simulink model "SecondaryPath_ANC"  (R2020a)
settings: Solver=FixedStepDiscrete  StartTime=0.0  StopTime=3  FixedStep=0.00025  RelTol=1e-3
libraries: dspsrcs4 x1, dspadpt3 x1
settings Model: Creator=The MathWorks, Inc.  LastModifiedBy=bruno
settings DataIOCC: ReturnWorkspaceOutputs=off
settings DebuggingCC: ArithmeticOperatorsInVariantConditions=warning
settings SFSimCC: CustomCodeUndefinedFunction=UseInterfaceOnly

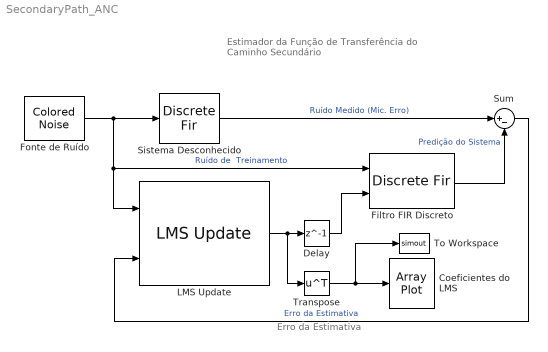
== system SecondaryPath_ANC ==
  note: Erro da Estimativa
  note: Estimador da Função de Transferência do
      | Caminho Secundário
  Coeficientes do LMS : ArrayPlot
  Delay : Delay  DelayLength=1
  Filtro FIR Discreto : DiscreteFir  CoefSource=Input port
      settings: InputPortMap=u0,u1
  Fonte de Ruído : dspsrcs4/Colored Noise  Color=white  InverseFrequencyPower=1  BoundedOutput=off  NumChannels=1  OutputDataType=double  SamplesPerFrame=1  SampleTime=1/4000  RandomStream=mt19937ar with seed  Seed=67  SimulateUsing=Interpreted execution
      settings: SourceProductBaseCode=DS
  LMS Update : dspadpt3/LMS Update  Method=Normalized LMS  Length=30  StepSizeSource=Property  StepSize=0.2  LeakageFactor=1.0  InitialConditions=0  EnableAdaptInput=off  EnableResetInput=off  SimulateUsing=Interpreted execution
      settings: SourceProductBaseCode=DS
  Sistema Desconhecido : DiscreteFir  Coefficients=[0.5 0.5 -.3 -.3 -.2 -.2 1 .7 -1.2 4]  InputProcessing=Columns as channels (frame based)
  Sum : Sum  Inputs=|+-
  To Workspace : ToWorkspace  VariableName=simout  SaveFormat=Timeseries  SampleTime=-1
  Transpose : Math  Operator=transpose  SignedPower=on  SaturateOnIntegerOverflow=on
  wires:
  Transpose/1 -> To Workspace/1, Coeficientes do LMS/1
  Sum/1 -> LMS Update/2  "Erro da Estimativa"
  Filtro FIR Discreto/1 -> Sum/2  "Predição do Sistema"
  Fonte de Ruído/1 -> Filtro FIR Discreto/1, LMS Update/1, Sistema Desconhecido/1  "Ruído de  Treinamento"
  LMS Update/1 -> Delay/1, Transpose/1
  Sistema Desconhecido/1 -> Sum/1  "Ruído Medido (Mic. Erro)"
  Delay/1 -> Filtro FIR Discreto/2
